simulink model "Kalman_Filter_vs_SS_Feedback_Control"  (R2018a)
settings: Solver=VariableStepAuto  StartTime=0.0  StopTime=10.0  RelTol=1e-3
settings Model: Creator=Rosa Garrido  LastModifiedBy=Rosa Garrido

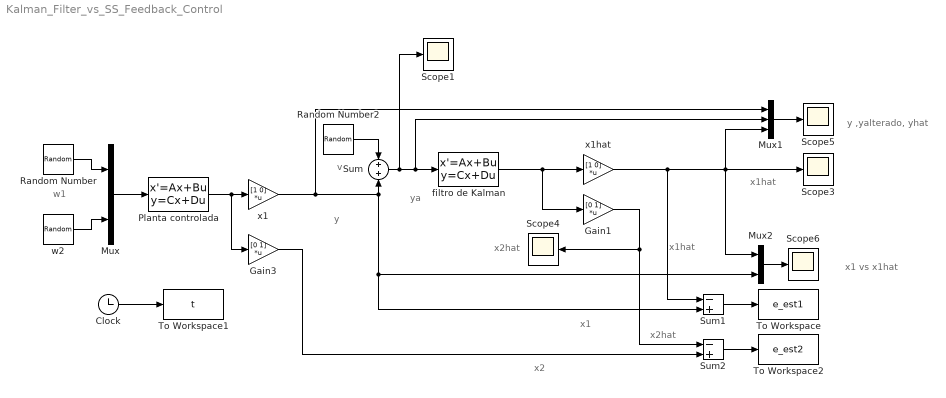
== system Kalman_Filter_vs_SS_Feedback_Control ==
  note: x2hat
  note: y ,yalterado, yhat
  note: x1 vs x1hat
  note: x1hat
  note: x1
  note: x2
  note: x2hat
  note: v
  note: ya
  note: y
  note: w1
  note: x1hat
  " w2" : RandomNumber  Variance=0.025  SampleTime=1e-3
  Clock : Clock
  Gain1 : Gain  Gain="[0  1]"  Multiplication=Matrix(K*u)
  Gain3 : Gain  Gain="[0  1]"  Multiplication=Matrix(K*u)
  Mux : Mux  Inputs=2
  Mux1 : Mux  Inputs=3
  Mux2 : Mux  Inputs=2
  Planta controlada : StateSpace  A="[ 0  1;  -2 -2]"  B="[0  0 ; -2  -1]"  C=eye(2)  D=zeros(2)  InitialCondition="[0.1  0]'"
  Random Number : RandomNumber  Variance=0.0025  SampleTime=1e-3
  Random Number2 : RandomNumber  Variance=0.25e-2  SampleTime=1e-3
  Scope{1,3..6} (5 alike) : Scope
  Sum : Sum
  Sum1 : Sum  Inputs=-+
  Sum2 : Sum  Inputs=-+
  To Workspace : ToWorkspace  VariableName=e_est1  SampleTime=-1
  To Workspace1 : ToWorkspace  VariableName=t  SampleTime=-1
  To Workspace2 : ToWorkspace  VariableName=e_est2  SampleTime=-1
  filtro de Kalman : StateSpace  A="[ -1.2532    1;  -2.7852 -2]"  B="[1.2532;  0.7852]"  C=eye(2)  D=zeros(2,1)  InitialCondition="[0  0]'"
  x1 : Gain  Gain=[1 0]  Multiplication=Matrix(K*u) (u vector)
  x1hat : Gain  Gain=[1 0]  Multiplication=Matrix(K*u)
  wires:
  Random Number/1 -> Mux/1
  " w2"/1 -> Mux/2
  Mux/1 -> Planta controlada/1
  Random Number2/1 -> Sum/1
  Planta controlada/1 -> x1/1, Gain3/1
  filtro de Kalman/1 -> x1hat/1, Gain1/1
  x1hat/1 -> Scope3/1, Mux1/3, Mux2/1, Sum1/1
  Gain1/1 -> Sum2/1, Scope4/1
  Mux1/1 -> Scope5/1
  Sum1/1 -> To Workspace/1
  Clock/1 -> To Workspace1/1
  Mux2/1 -> Scope6/1
  Gain3/1 -> Sum2/2
  Sum2/1 -> To Workspace2/1
  x1/1 -> Mux1/1, Mux2/2, Sum1/2, Sum/2
  Sum/1 -> Scope1/1, Mux1/2, filtro de Kalman/1
